simulink subsystem "PvtSubSys_PLAN_DPC"  (R2020b)
settings: Solver=VariableStepAuto  StartTime=0.0  StopTime=10.0  RelTol=1e-3
undefined symbols (not defined in the file or in its folder): P_Global_DxvFrontBumper_m, P_Global_DxvRearBumper_m, P_PLAN_DPC_BrkPointDxFactorF1, P_PLAN_DPC_BrkPointDxFactorF2, P_PLAN_DPC_BrkPointDxFactorF3, P_PLAN_DPC_BrkPointDxFactorF4, P_PLAN_DPC_BrkPointDxFactorR1, P_PLAN_DPC_BrkPointDxFactorR2, P_PLAN_DPC_BrkPointDxFactorR3, P_PLAN_DPC_BrkPointDxFactorR4, P_PLAN_DPC_danqianleida_kaiguan, P_PLAN_DPC_danqianleida_maxDx, P_PLAN_DPC_danqianleida_minDx, P_PLAN_DPC_FrontObj_DX_00, P_PLAN_DPC_FrontObj_DX_03, P_PLAN_DPC_FrontObj_DX_08, P_PLAN_DPC_FrontObj_DX_1, P_PLAN_DPC_HearObj_DX_00, P_PLAN_DPC_HearObj_DX_03, P_PLAN_DPC_HearObj_DX_08, P_PLAN_DPC_HearObj_DX_11, P_PLAN_DPC_HWALineRearA2Factor, P_PLAN_DPC_HWALineRearA3Factor, P_PLAN_DPC_ObjAxLPalpha, P_PLAN_DPC_ObjDxLPalpha, P_PLAN_DPC_ObjDyLPalpha, P_PLAN_DPC_ObjVxLPalpha, P_PLAN_DPC_xiangduisudu_kmh
libraries: simulink x22
(part 2 of 3)

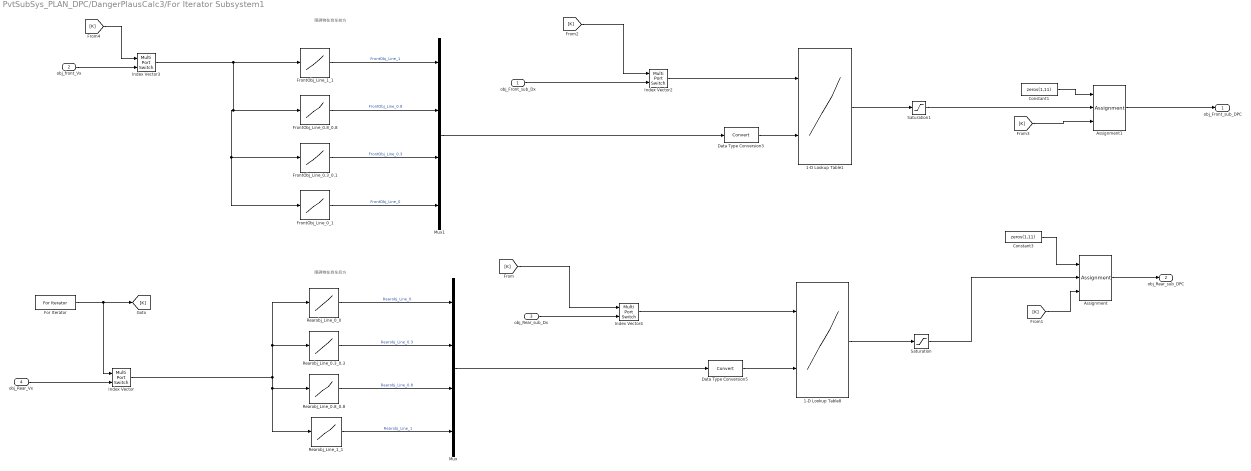
== system PvtSubSys_PLAN_DPC/DangerPlausCalc3/For Iterator Subsystem1 ==
  note: 障碍物在自车后方
  note: 障碍物在自车前方
  obj_Front_sub_Dx : Inport
  obj_front_Vx : Inport  Port=2
  obj_Rear_sub_Dx : Inport  Port=3
  obj_Rear_Vx : Inport  Port=4
  1-D Lookup Table1 : Lookup_n-D  NumberOfTableDimensions=1  BreakpointsForDimension1Source=Input port  BreakpointsForDimension1=[-5:5]  Table=[1 0.8 0.3 0]  InternalRulePriority=Speed  RndMeth=Simplest  InputSameDT=on
      settings: InputPortMap=u0,p5
  1-D Lookup Table8 : Lookup_n-D  NumberOfTableDimensions=1  BreakpointsForDimension1Source=Input port  BreakpointsForDimension1=[-5:5]  Table=[0 0.3 0.8 1]  InternalRulePriority=Speed  RndMeth=Simplest  InputSameDT=on
      settings: InputPortMap=u0,p5
  Assignment : Assignment  DiagnosticForDimensions=Warning  IndexOptions=Index vector (port)  Indices=1  OutputSizes=1
  Assignment1 : Assignment  DiagnosticForDimensions=Warning  IndexOptions=Index vector (port)  Indices=1  OutputSizes=1
  Constant1 : Constant  Value=zeros(1,11)  OutDataTypeStr=single
  Constant3 : Constant  Value=zeros(1,11)  OutDataTypeStr=single
  Data Type Conversion3 : DataTypeConversion
  Data Type Conversion5 : DataTypeConversion
  For Iterator : ForIterator  ResetStates=reset  IterationLimit=11  IterationVariableDataType=int8
  FrontObj_Line_0.3_0.1 : Lookup_n-D  NumberOfTableDimensions=1  BreakpointsForDimension1="[-49.5\t-33\t-18\t-16.5\t-7\t-6\t-2.5\t-2\t-1.5\t-0.5\t0\t0.5\t1.5\t4\t4.5\t5\t5.5\t7\t9.5\t10\t12.5\t18.5\t30]"  Table="[160\t112\t64\t60\t26.4\t23.6\t19\t18.4\t17.8\t16.6\t16.2\t15.6\t14.6\t13\t12.8\t12.4\t12.2\t11.8\t11.2\t11\t10.6\t9.2\t9.2]"  InternalRulePriority=Speed  RndMeth=Simplest  InputSameDT=on
  FrontObj_Line_0.8_0.8 : Lookup_n-D  NumberOfTableDimensions=1  BreakpointsForDimension1="[-49.5\t-33\t-18\t-16.5\t-7\t-6\t-2.5\t-2\t-1.5\t-0.5\t0\t0.5\t1.5\t4\t4.5\t5\t5.5\t7\t9.5\t10\t12.5\t18.5\t30]"  Table="[82\t58\t31.2\t29.2\t16\t14.8\t11\t10.4\t9.8\t8.6\t8.2\t7.6\t7.6\t7.6\t7.6\t7.6\t7.6\t7.6\t7.6\t7.6\t7.6\t7.6\t7.6]"  InternalRulePriority=Speed  RndMeth=Simplest  InputSameDT=on
  FrontObj_Line_0_1 : Lookup_n-D  NumberOfTableDimensions=1  BreakpointsForDimension1="[-49.5\t-33\t-18\t-16.5\t-7\t-6\t-2.5\t-2\t-1.5\t-0.5\t0\t0.5\t1.5\t4\t4.5\t5\t5.5\t7\t9.5\t10\t12.5\t18.5\t30]"  Table="[215\t150\t89\t82\t36.4\t32.4\t23.8\t23.2\t22.6\t21.6\t21\t20.4\t19.2\t16.6\t16\t15.4\t15.2\t14.4\t13.2\t13.2\t12.4\t11.2\t11.2]"  InternalRulePriority=Speed  RndMeth=Simplest  InputSameDT=on
  FrontObj_Line_1_1 : Lookup_n-D  NumberOfTableDimensions=1  BreakpointsForDimension1="[-49.5\t-33\t-18\t-16.5\t-7\t-6\t-2.5\t-2\t-1.5\t-0.5\t0\t0.5\t1.5\t4\t4.5\t5\t5.5\t7\t9.5\t10\t12.5\t18.5\t30]"  Table="[68\t46\t26.2\t24.4\t14\t12.8\t9\t8.4\t7.8\t6.6\t6.2\t5.6\t5.6\t5.6\t5.6\t5.6\t5.6\t5.6\t5.6\t5.6\t5.6\t5.6\t5.6]"  ExtrapMethod=Clip  UseLastTableValue=on  InternalRulePriority=Speed  RndMeth=Simplest  InputSameDT=on
  Index Vector : MultiPortSwitch  Inputs=1
  Index Vector2 : MultiPortSwitch  Inputs=1  OutDataTypeStr=single
  Index Vector3 : MultiPortSwitch  Inputs=1
  Index Vector4 : MultiPortSwitch  Inputs=1  OutDataTypeStr=single
  Mux : Mux
  Mux1 : Mux
  Rearobj_Line_0.3_0.3 : Lookup_n-D  NumberOfTableDimensions=1  BreakpointsForDimension1="[-49.5\t-33\t-18\t-16.5\t-7\t-6\t-2.5\t-2\t-1.5\t-0.5\t0\t0.5\t1.5\t4\t4.5\t5\t5.5\t7\t9.5\t10\t12.5\t18.5\t30]"  Table="[-2.7\t-3.4\t-4.6\t-4.8\t-6.6\t-7\t-8.8\t-9\t-9.4\t-10.2\t-10.8\t-11.2\t-12.4\t-15.2\t-15.6\t-16.2\t-16.8\t-18.4\t-24.2\t-25.6\t-32.4\t-48.5\t-76.4]"  InternalRulePriority=Speed  RndMeth=Simplest  InputSameDT=on
  Rearobj_Line_0.8_0.8 : Lookup_n-D  NumberOfTableDimensions=1  BreakpointsForDimension1="[-49.5\t-33\t-18\t-16.5\t-7\t-6\t-2.5\t-2\t-1.5\t-0.5\t0\t0.5\t1.5\t4\t4.5\t5\t5.5\t7\t9.5\t10\t12.5\t18.5\t30]"  Table="[-1.19\t-1.2\t-1.2\t-1.2\t-1.2\t-1.2\t-1.2\t-1.2\t-1.2\t-1.2\t-1.2\t-1.2\t-2.4\t-5.2\t-5.6\t-6.2\t-6.8\t-8.4\t-11.8\t-12.4\t-16\t-24.2\t-38]"  InternalRulePriority=Speed  RndMeth=Simplest  InputSameDT=on
  Rearobj_Line_0_0 : Lookup_n-D  NumberOfTableDimensions=1  BreakpointsForDimension1="[-49.5\t-33\t-18\t-16.5\t-7\t-6\t-2.5\t-2\t-1.5\t-0.5\t0\t0.5\t1.5\t4\t4.5\t5\t5.5\t7\t9.5\t10\t12.5\t18.5\t30]"  Table="[-3.9\t-5\t-7\t-7.4\t-11\t-11.8\t-15.6\t-16.2\t-16.8\t-17.8\t-18.4\t-19\t-20\t-22.8\t-23.4\t-24\t-24.6\t-28.2\t-38.2\t-40.2\t-47.3\t-71\t-100]"  InternalRulePriority=Speed  RndMeth=Simplest  InputSameDT=on
  Rearobj_Line_1_1 : Lookup_n-D  NumberOfTableDimensions=1  BreakpointsForDimension1="[-49.5\t-33\t-18\t-16.5\t-7\t-6\t-2.5\t-2\t-1.5\t-0.5\t0\t0.5\t1.5\t4\t4.5\t5\t5.5\t7\t9.5\t10\t12.5\t18.5\t30]"  Table="[0.8\t0.8\t0.8\t0.8\t0.8\t0.8\t0.8\t0.8\t0.8\t0.8\t0.8\t0.8\t-0.4\t-3.2\t-3.6\t-4.2\t-4.8\t-6.4\t-9.2\t-9.8\t-12.6\t-19.2\t-30]"  InternalRulePriority=Speed  RndMeth=Simplest  InputSameDT=on
  Saturation : Saturate  UpperLimit=1  LowerLimit=0
  Saturation1 : Saturate  UpperLimit=1  LowerLimit=0
  obj_Front_sub_DPC : Outport
  obj_Rear_sub_DPC : Outport  Port=2
  wires:
  Data Type Conversion5/1 -> 1-D Lookup Table8/2
  Index Vector4/1 -> 1-D Lookup Table8/1
  Data Type Conversion3/1 -> 1-D Lookup Table1/2
  Index Vector2/1 -> 1-D Lookup Table1/1
  Saturation/1 -> Assignment/2
  Saturation1/1 -> Assignment1/2
  obj_front_Vx/1 -> Index Vector3/2
  Index Vector3/1 -> FrontObj_Line_1_1/1, FrontObj_Line_0_1/1, FrontObj_Line_0.3_0.1/1, FrontObj_Line_0.8_0.8/1
  [K] -> Index Vector3/1
  Assignment1/1 -> obj_Front_sub_DPC/1
  Constant1/1 -> Assignment1/1
  [K] -> Assignment1/3
  [K] -> Index Vector2/1
  Assignment/1 -> obj_Rear_sub_DPC/1
  [K] -> Assignment/3
  Constant3/1 -> Assignment/1
  [K] -> Index Vector4/1
  For Iterator/1 -> [K], Index Vector/1
  obj_Rear_Vx/1 -> Index Vector/2
  Rearobj_Line_0.3_0.3/1 -> Mux/2  "Rearobj_Line_0.3"
  Index Vector/1 -> Rearobj_Line_0.3_0.3/1, Rearobj_Line_0_0/1, Rearobj_Line_1_1/1, Rearobj_Line_0.8_0.8/1
  Mux1/1 -> Data Type Conversion3/1
  FrontObj_Line_0.8_0.8/1 -> Mux1/2  "FrontObj_Line_0.8"
  obj_Front_sub_Dx/1 -> Index Vector2/2
  FrontObj_Line_1_1/1 -> Mux1/1  "FrontObj_Line_1"
  1-D Lookup Table1/1 -> Saturation1/1
  Rearobj_Line_1_1/1 -> Mux/4  "Rearobj_Line_1"
  FrontObj_Line_0_1/1 -> Mux1/4  "FrontObj_Line_0"
  1-D Lookup Table8/1 -> Saturation/1
  Mux/1 -> Data Type Conversion5/1
  obj_Rear_sub_Dx/1 -> Index Vector4/2
  Rearobj_Line_0_0/1 -> Mux/1  "Rearobj_Line_0"
  FrontObj_Line_0.3_0.1/1 -> Mux1/3  "FrontObj_Line_0.3"
  Rearobj_Line_0.8_0.8/1 -> Mux/3  "Rearobj_Line_0.8"

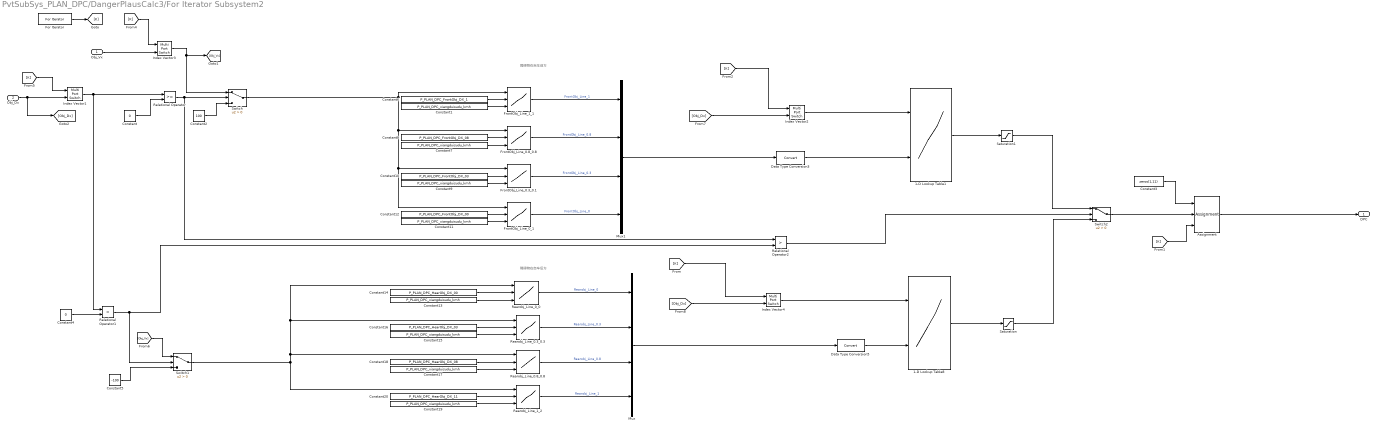
== system PvtSubSys_PLAN_DPC/DangerPlausCalc3/For Iterator Subsystem2 ==
  note: 障碍物在自车后方
  note: 障碍物在自车前方
  Obj_Vx : Inport
  Obj_Dx : Inport  Port=2
  1-D Lookup Table1 : Lookup_n-D  NumberOfTableDimensions=1  BreakpointsForDimension1Source=Input port  BreakpointsForDimension1=[-5:5]  Table=[1 0.8 0.3 0]  ExtrapMethod=Clip  InternalRulePriority=Speed  RndMeth=Simplest  InputSameDT=on
      settings: InputPortMap=u0,p5
  1-D Lookup Table8 : Lookup_n-D  NumberOfTableDimensions=1  BreakpointsForDimension1Source=Input port  BreakpointsForDimension1=[-5:5]  Table=[0 0.3 0.8 1]  ExtrapMethod=Clip  InternalRulePriority=Speed  RndMeth=Simplest  InputSameDT=on
      settings: InputPortMap=u0,p5
  Assignment : Assignment  DiagnosticForDimensions=Warning  IndexOptions=Index vector (port)  Indices=1  OutputSizes=1
  Constant : Constant  Value=0  OutDataTypeStr=single
  Constant{1,7,9,11,13,15,17,19} (8 alike) : Constant  Value=P_PLAN_DPC_xiangduisudu_kmh  OutDataTypeStr=single
  Constant10 : Constant  Value=P_PLAN_DPC_FrontObj_DX_03  OutDataTypeStr=single
  Constant12 : Constant  Value=P_PLAN_DPC_FrontObj_DX_00  OutDataTypeStr=single
  Constant14 : Constant  Value=P_PLAN_DPC_HearObj_DX_00  OutDataTypeStr=single
  Constant16 : Constant  Value=P_PLAN_DPC_HearObj_DX_03  OutDataTypeStr=single
  Constant18 : Constant  Value=P_PLAN_DPC_HearObj_DX_08  OutDataTypeStr=single
  Constant2 : Constant  Value=100  OutDataTypeStr=single
  Constant20 : Constant  Value=P_PLAN_DPC_HearObj_DX_11  OutDataTypeStr=single
  Constant3 : Constant  Value=zeros(1,11)  OutDataTypeStr=single
  Constant4 : Constant  Value=0  OutDataTypeStr=single
  Constant5 : Constant  Value=-100  OutDataTypeStr=single
  Constant6 : Constant  Value=P_PLAN_DPC_FrontObj_DX_1  OutDataTypeStr=single
  Constant8 : Constant  Value=P_PLAN_DPC_FrontObj_DX_08  OutDataTypeStr=single
  Data Type Conversion3 : DataTypeConversion
  Data Type Conversion5 : DataTypeConversion
  For Iterator : ForIterator  ResetStates=reset  IterationLimit=11  IterationVariableDataType=int8
  FrontObj_Line_0.3_0.1 : Lookup_n-D  NumberOfTableDimensions=1  BreakpointsForDimension1Source=Input port  BreakpointsForDimension1="[-49.5\t-33\t-18\t-16.5\t-7\t-6\t-2.5\t-2\t-1.5\t-0.5\t0\t0.5\t1.5\t4\t4.5\t5\t5.5\t7\t9.5\t10\t12.5\t18.5\t30 50]"  TableSource=Input port  Table="[160\t112\t64\t60\t26.4\t23.6\t19\t18.4\t17.8\t16.6\t16.2\t15.6\t14.6\t13\t12.8\t12.4\t12.2\t11.8\t11.2\t11\t10.6\t9.2\t9.2 9.2]"  InternalRulePriority=Speed  RndMeth=Simplest  InputSameDT=on
      settings: InputPortMap=u0,p221,p5
  FrontObj_Line_0.8_0.8 : Lookup_n-D  NumberOfTableDimensions=1  BreakpointsForDimension1Source=Input port  BreakpointsForDimension1="[-49.5\t-33\t-18\t-16.5\t-7\t-6\t-2.5\t-2\t-1.5\t-0.5\t0\t0.5\t1.5\t4\t4.5\t5\t5.5\t7\t9.5\t10\t12.5\t18.5\t30 50]"  TableSource=Input port  Table="[82\t58\t31.2\t29.2\t16\t14.8\t11\t10.4\t9.8\t8.6\t8.2\t7.6\t7.6\t7.6\t7.6\t7.6\t7.6\t7.6\t7.6\t7.6\t7.6\t7.6\t7.6 7.6]"  InternalRulePriority=Speed  RndMeth=Simplest  InputSameDT=on
      settings: InputPortMap=u0,p221,p5
  FrontObj_Line_0_1 : Lookup_n-D  NumberOfTableDimensions=1  BreakpointsForDimension1Source=Input port  BreakpointsForDimension1="[-49.5\t-33\t-18\t-16.5\t-7\t-6\t-2.5\t-2\t-1.5\t-0.5\t0\t0.5\t1.5\t4\t4.5\t5\t5.5\t7\t9.5\t10\t12.5\t18.5\t30 50]"  TableSource=Input port  Table="[215\t150\t89\t82\t36.4\t32.4\t23.8\t23.2\t22.6\t21.6\t21\t20.4\t19.2\t16.6\t16\t15.4\t15.2\t14.4\t13.2\t13.2\t12.4\t11.2\t11.2 11.2]"  InternalRulePriority=Speed  RndMeth=Simplest  InputSameDT=on
      settings: InputPortMap=u0,p221,p5
  FrontObj_Line_1_1 : Lookup_n-D  NumberOfTableDimensions=1  BreakpointsForDimension1Source=Input port  BreakpointsForDimension1="[-49.5\t-33\t-18\t-16.5\t-7\t-6\t-2.5\t-2\t-1.5\t-0.5\t0\t0.5\t1.5\t4\t4.5\t5\t5.5\t7\t9.5\t10\t12.5\t18.5\t30 50]"  TableSource=Input port  Table="[68\t      46\t26.2\t24.4\t14\t    12.8\t9\t    8.4 \t7.8\t     6.6\t6.2\t     5.6\t5.6 \t5.6\t     5.6\t5.6\t     5.6\t5.6\t    5.6\t    5.6     5.6\t     5.6\t5.6  5.6]"  UseLastTableValue=on  InternalRulePriority=Speed  RndMeth=Simplest  InputSameDT=on
      settings: InputPortMap=u0,p221,p5
  Index Vector1 : MultiPortSwitch  Inputs=1
  Index Vector2 : MultiPortSwitch  Inputs=1  OutDataTypeStr=single
  Index Vector3 : MultiPortSwitch  Inputs=1
  Index Vector4 : MultiPortSwitch  Inputs=1  OutDataTypeStr=single
  Mux : Mux
  Mux1 : Mux
  Rearobj_Line_0.3_0.3 : Lookup_n-D  NumberOfTableDimensions=1  BreakpointsForDimension1Source=Input port  BreakpointsForDimension1="[-49.5\t-33\t-18\t-16.5\t-7\t-6\t-2.5\t-2\t-1.5\t-0.5\t0\t0.5\t1.5\t4\t4.5\t5\t5.5\t7\t9.5\t10\t12.5\t18.5\t30 50]"  TableSource=Input port  Table="[-7   \t-7  \t-7  \t-7  \t-7  \t-7  \t -8.1 \t-9  \t-9.4  \t-10.2\t-10.8\t-11.2\t-12.4\t-15.2\t-15.6\t-16.2\t-16.8\t-19.4\t-24.2\t-25.6\t-30.4\t-48.5\t-86.4 -140]"  InternalRulePriority=Speed  RndMeth=Simplest  InputSameDT=on
      settings: InputPortMap=u0,p221,p5
  Rearobj_Line_0.8_0.8 : Lookup_n-D  NumberOfTableDimensions=1  BreakpointsForDimension1Source=Input port  BreakpointsForDimension1="[-49.5\t-33\t-18\t-16.5\t-7\t-6\t-2.5\t-2\t-1.5\t-0.5\t0\t0.5\t1.5\t4\t4.5\t5\t5.5\t7\t9.5\t10\t12.5\t18.5\t30 50]"  TableSource=Input port  Table="[-2.4    -2.4\t    -2.4\t-2.4\t-2.4\t-2.4\t-2.4\t-2.4\t-2.4\t-2.4\t-2.4\t-2.4\t-2.4\t-5.2\t-5.6\t-6.2\t  -6.8   \t-8.4\t-11.8\t-12.4\t-16\t    -24.2\t-38 -60]"  InternalRulePriority=Speed  RndMeth=Simplest  InputSameDT=on
      settings: InputPortMap=u0,p221,p5
  Rearobj_Line_0_0 : Lookup_n-D  NumberOfTableDimensions=1  BreakpointsForDimension1Source=Input port  BreakpointsForDimension1="[-49.5\t-33\t-18\t-16.5\t-7\t-6\t-2.5\t-2\t-1.5\t-0.5\t0\t0.5\t1.5\t4\t4.5\t5\t5.5\t7\t9.5\t10\t12.5\t18.5\t30 50]"  TableSource=Input port  Table="[-13\t     -13\t -13    -13 \t-13\t    -14\t    -15.6\t-16.2\t-16.8\t-17.8\t-18.4\t-19  \t-20  \t-22.8\t-23.4\t-24\t    -24.6\t-28.2\t-38.2\t-40.2\t-47.3\t-68\t    -100 -160]"  InternalRulePriority=Speed  RndMeth=Simplest  InputSameDT=on
      settings: InputPortMap=u0,p221,p5
  Rearobj_Line_1_2 : Lookup_n-D  NumberOfTableDimensions=1  BreakpointsForDimension1Source=Input port  BreakpointsForDimension1="[-49.5\t-33\t-18\t-16.5\t-7\t-6\t-2.5\t-2\t-1.5\t-0.5\t0\t0.5\t1.5\t4\t4.5\t5\t5.5\t7\t9.5\t10\t12.5\t18.5\t30 50]"  TableSource=Input port  Table="[-2\t     -2 \t-2\t    -2\t    -2 \t    -2    \t-2\t   -2 \t   -2\t    -2\t    -2      -2\t   -2       -3.2\t -3.6\t -4.2\t -4.8\t -6.4\t -9.2\t   -9.8\t   -12.6\t-19.2\t-30 -30]"  InternalRulePriority=Speed  RndMeth=Simplest  InputSameDT=on
      settings: InputPortMap=u0,p221,p5
  Relational Operator : RelationalOperator  OutDataTypeStr=boolean  RndMeth=Simplest
  Relational Operator1 : RelationalOperator  Operator=<  OutDataTypeStr=boolean  RndMeth=Simplest
  Relational Operator2 : RelationalOperator  Operator=>  OutDataTypeStr=boolean  RndMeth=Simplest
  Saturation : Saturate  UpperLimit=1  LowerLimit=0
  Saturation1 : Saturate  UpperLimit=1  LowerLimit=0
  Switch : Switch  Criteria=u2 > Threshold
  Switch1 : Switch  Criteria=u2 > Threshold
  Switch2 : Switch  Criteria=u2 > Threshold
  DPC : Outport
  wires:
  Constant19/1 -> Rearobj_Line_1_2/3
  Constant13/1 -> Rearobj_Line_0_0/3
  Constant18/1 -> Rearobj_Line_0.8_0.8/2
  Constant17/1 -> Rearobj_Line_0.8_0.8/3
  Constant14/1 -> Rearobj_Line_0_0/2
  Constant15/1 -> Rearobj_Line_0.3_0.3/3
  Switch1/1 -> Rearobj_Line_1_2/1, Rearobj_Line_0_0/1, Rearobj_Line_0.3_0.3/1, Rearobj_Line_0.8_0.8/1
  Constant20/1 -> Rearobj_Line_1_2/2
  Constant16/1 -> Rearobj_Line_0.3_0.3/2
  Switch/1 -> FrontObj_Line_0.8_0.8/1, FrontObj_Line_0.3_0.1/1, FrontObj_Line_0_1/1, FrontObj_Line_1_1/1
  Constant1/1 -> FrontObj_Line_1_1/3
  Constant8/1 -> FrontObj_Line_0.8_0.8/2
  Constant6/1 -> FrontObj_Line_1_1/2
  Constant9/1 -> FrontObj_Line_0.3_0.1/3
  Constant10/1 -> FrontObj_Line_0.3_0.1/2
  Constant11/1 -> FrontObj_Line_0_1/3
  Constant7/1 -> FrontObj_Line_0.8_0.8/3
  Constant12/1 -> FrontObj_Line_0_1/2
  Index Vector4/1 -> 1-D Lookup Table8/1
  Index Vector2/1 -> 1-D Lookup Table1/1
  Saturation/1 -> Switch2/3
  Saturation1/1 -> Switch2/1
  Switch2/1 -> Assignment/2
  Relational Operator2/1 -> Switch2/2
  Assignment/1 -> DPC/1
  [Obj_Dx] -> Index Vector4/2
  [Obj_Dx] -> Index Vector2/2
  Constant5/1 -> Switch1/3
  [Obj_Vx] -> Switch1/1
  Index Vector3/1 -> Switch/1, [Obj_Vx]
  Relational Operator1/1 -> Switch1/2, Relational Operator2/2
  Constant4/1 -> Relational Operator1/2
  Constant2/1 -> Switch/3
  Relational Operator/1 -> Switch/2, Relational Operator2/1
  Constant/1 -> Relational Operator/2
  Index Vector1/1 -> Relational Operator1/1, Relational Operator/1
  [K] -> Index Vector1/1
  Obj_Dx/1 -> Index Vector1/2, [Obj_Dx]
  Obj_Vx/1 -> Index Vector3/2
  Data Type Conversion5/1 -> 1-D Lookup Table8/2
  Data Type Conversion3/1 -> 1-D Lookup Table1/2
  [K] -> Index Vector3/1
  [K] -> Index Vector2/1
  [K] -> Assignment/3
  Constant3/1 -> Assignment/1
  [K] -> Index Vector4/1
  For Iterator/1 -> [K]
  Rearobj_Line_0.3_0.3/1 -> Mux/2  "Rearobj_Line_0.3"
  Mux1/1 -> Data Type Conversion3/1
  FrontObj_Line_0.8_0.8/1 -> Mux1/2  "FrontObj_Line_0.8"
  FrontObj_Line_1_1/1 -> Mux1/1  "FrontObj_Line_1"
  1-D Lookup Table1/1 -> Saturation1/1
  Rearobj_Line_1_2/1 -> Mux/4  "Rearobj_Line_1"
  FrontObj_Line_0_1/1 -> Mux1/4  "FrontObj_Line_0"
  1-D Lookup Table8/1 -> Saturation/1
  Mux/1 -> Data Type Conversion5/1
  Rearobj_Line_0_0/1 -> Mux/1  "Rearobj_Line_0"
  FrontObj_Line_0.3_0.1/1 -> Mux1/3  "FrontObj_Line_0.3"
  Rearobj_Line_0.8_0.8/1 -> Mux/3  "Rearobj_Line_0.8"

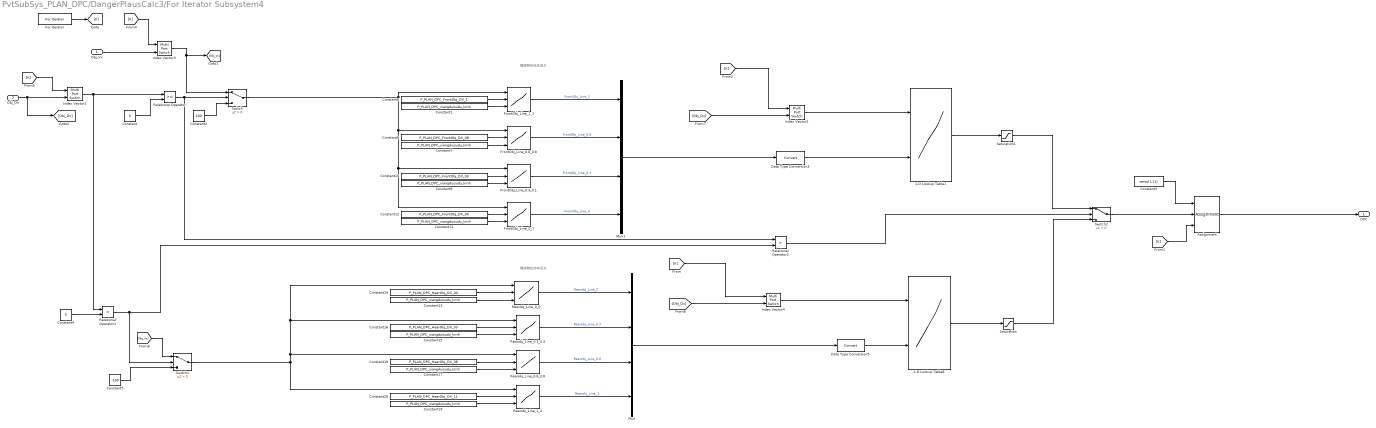
== system PvtSubSys_PLAN_DPC/DangerPlausCalc3/For Iterator Subsystem4 ==
  note: 障碍物在自车前方
  note: 障碍物在自车后方
  Obj_Vx : Inport
  Obj_Dx : Inport  Port=2
  1-D Lookup Table1 : Lookup_n-D  NumberOfTableDimensions=1  BreakpointsForDimension1Source=Input port  BreakpointsForDimension1=[-5:5]  Table=[1 0.8 0.3 0]  ExtrapMethod=Clip  InternalRulePriority=Speed  RndMeth=Simplest  InputSameDT=on
      settings: InputPortMap=u0,p5
  1-D Lookup Table8 : Lookup_n-D  NumberOfTableDimensions=1  BreakpointsForDimension1Source=Input port  BreakpointsForDimension1=[-5:5]  Table=[0 0.3 0.8 1]  ExtrapMethod=Clip  InternalRulePriority=Speed  RndMeth=Simplest  InputSameDT=on
      settings: InputPortMap=u0,p5
  Assignment : Assignment  DiagnosticForDimensions=Warning  IndexOptions=Index vector (port)  Indices=1  OutputSizes=1
  Constant : Constant  Value=0  OutDataTypeStr=single
  Constant{1,7,9,11,13,15,17,19} (8 alike) : Constant  Value=P_PLAN_DPC_xiangduisudu_kmh  OutDataTypeStr=single
  Constant10 : Constant  Value=P_PLAN_DPC_FrontObj_DX_03  OutDataTypeStr=single
  Constant12 : Constant  Value=P_PLAN_DPC_FrontObj_DX_00  OutDataTypeStr=single
  Constant14 : Constant  Value=P_PLAN_DPC_HearObj_DX_00  OutDataTypeStr=single
  Constant16 : Constant  Value=P_PLAN_DPC_HearObj_DX_03  OutDataTypeStr=single
  Constant18 : Constant  Value=P_PLAN_DPC_HearObj_DX_08  OutDataTypeStr=single
  Constant2 : Constant  Value=100  OutDataTypeStr=single
  Constant20 : Constant  Value=P_PLAN_DPC_HearObj_DX_11  OutDataTypeStr=single
  Constant3 : Constant  Value=zeros(1,11)  OutDataTypeStr=single
  Constant4 : Constant  Value=0  OutDataTypeStr=single
  Constant5 : Constant  Value=-100  OutDataTypeStr=single
  Constant6 : Constant  Value=P_PLAN_DPC_FrontObj_DX_1  OutDataTypeStr=single
  Constant8 : Constant  Value=P_PLAN_DPC_FrontObj_DX_08  OutDataTypeStr=single
  Data Type Conversion3 : DataTypeConversion
  Data Type Conversion5 : DataTypeConversion
  For Iterator : ForIterator  ResetStates=reset  IterationLimit=11  IterationVariableDataType=int8
  FrontObj_Line_0.3_0.1 : Lookup_n-D  NumberOfTableDimensions=1  BreakpointsForDimension1Source=Input port  BreakpointsForDimension1="[-49.5\t-33\t-18\t-16.5\t-7\t-6\t-2.5\t-2\t-1.5\t-0.5\t0\t0.5\t1.5\t4\t4.5\t5\t5.5\t7\t9.5\t10\t12.5\t18.5\t30 50]"  TableSource=Input port  Table="[160\t112\t64\t60\t26.4\t23.6\t19\t18.4\t17.8\t16.6\t16.2\t15.6\t14.6\t13\t12.8\t12.4\t12.2\t11.8\t11.2\t11\t10.6\t9.2\t9.2 9.2]"  InternalRulePriority=Speed  RndMeth=Simplest  InputSameDT=on
      settings: InputPortMap=u0,p221,p5
  FrontObj_Line_0.8_0.8 : Lookup_n-D  NumberOfTableDimensions=1  BreakpointsForDimension1Source=Input port  BreakpointsForDimension1="[-49.5\t-33\t-18\t-16.5\t-7\t-6\t-2.5\t-2\t-1.5\t-0.5\t0\t0.5\t1.5\t4\t4.5\t5\t5.5\t7\t9.5\t10\t12.5\t18.5\t30 50]"  TableSource=Input port  Table="[82\t58\t31.2\t29.2\t16\t14.8\t11\t10.4\t9.8\t8.6\t8.2\t7.6\t7.6\t7.6\t7.6\t7.6\t7.6\t7.6\t7.6\t7.6\t7.6\t7.6\t7.6 7.6]"  InternalRulePriority=Speed  RndMeth=Simplest  InputSameDT=on
      settings: InputPortMap=u0,p221,p5
  FrontObj_Line_0_1 : Lookup_n-D  NumberOfTableDimensions=1  BreakpointsForDimension1Source=Input port  BreakpointsForDimension1="[-49.5\t-33\t-18\t-16.5\t-7\t-6\t-2.5\t-2\t-1.5\t-0.5\t0\t0.5\t1.5\t4\t4.5\t5\t5.5\t7\t9.5\t10\t12.5\t18.5\t30 50]"  TableSource=Input port  Table="[215\t150\t89\t82\t36.4\t32.4\t23.8\t23.2\t22.6\t21.6\t21\t20.4\t19.2\t16.6\t16\t15.4\t15.2\t14.4\t13.2\t13.2\t12.4\t11.2\t11.2 11.2]"  InternalRulePriority=Speed  RndMeth=Simplest  InputSameDT=on
      settings: InputPortMap=u0,p221,p5
  FrontObj_Line_1_1 : Lookup_n-D  NumberOfTableDimensions=1  BreakpointsForDimension1Source=Input port  BreakpointsForDimension1="[-49.5\t-33\t-18\t-16.5\t-7\t-6\t-2.5\t-2\t-1.5\t-0.5\t0\t0.5\t1.5\t4\t4.5\t5\t5.5\t7\t9.5\t10\t12.5\t18.5\t30 50]"  TableSource=Input port  Table="[68\t      46\t26.2\t24.4\t14\t    12.8\t9\t    8.4 \t7.8\t     6.6\t6.2\t     5.6\t5.6 \t5.6\t     5.6\t5.6\t     5.6\t5.6\t    5.6\t    5.6     5.6\t     5.6\t5.6  5.6]"  UseLastTableValue=on  InternalRulePriority=Speed  RndMeth=Simplest  InputSameDT=on
      settings: InputPortMap=u0,p221,p5
  Index Vector1 : MultiPortSwitch  Inputs=1
  Index Vector2 : MultiPortSwitch  Inputs=1  OutDataTypeStr=single
  Index Vector3 : MultiPortSwitch  Inputs=1
  Index Vector4 : MultiPortSwitch  Inputs=1  OutDataTypeStr=single
  Mux : Mux
  Mux1 : Mux
  Rearobj_Line_0.3_0.3 : Lookup_n-D  NumberOfTableDimensions=1  BreakpointsForDimension1Source=Input port  BreakpointsForDimension1="[-49.5\t-33\t-18\t-16.5\t-7\t-6\t-2.5\t-2\t-1.5\t-0.5\t0\t0.5\t1.5\t4\t4.5\t5\t5.5\t7\t9.5\t10\t12.5\t18.5\t30 50]"  TableSource=Input port  Table="[-7   \t-7  \t-7  \t-7  \t-7  \t-7  \t -8.1 \t-9  \t-9.4  \t-10.2\t-10.8\t-11.2\t-12.4\t-15.2\t-15.6\t-16.2\t-16.8\t-19.4\t-24.2\t-25.6\t-30.4\t-48.5\t-86.4 -140]"  InternalRulePriority=Speed  RndMeth=Simplest  InputSameDT=on
      settings: InputPortMap=u0,p221,p5
  Rearobj_Line_0.8_0.8 : Lookup_n-D  NumberOfTableDimensions=1  BreakpointsForDimension1Source=Input port  BreakpointsForDimension1="[-49.5\t-33\t-18\t-16.5\t-7\t-6\t-2.5\t-2\t-1.5\t-0.5\t0\t0.5\t1.5\t4\t4.5\t5\t5.5\t7\t9.5\t10\t12.5\t18.5\t30 50]"  TableSource=Input port  Table="[-2.4    -2.4\t    -2.4\t-2.4\t-2.4\t-2.4\t-2.4\t-2.4\t-2.4\t-2.4\t-2.4\t-2.4\t-2.4\t-5.2\t-5.6\t-6.2\t  -6.8   \t-8.4\t-11.8\t-12.4\t-16\t    -24.2\t-38 -60]"  InternalRulePriority=Speed  RndMeth=Simplest  InputSameDT=on
      settings: InputPortMap=u0,p221,p5
  Rearobj_Line_0_0 : Lookup_n-D  NumberOfTableDimensions=1  BreakpointsForDimension1Source=Input port  BreakpointsForDimension1="[-49.5\t-33\t-18\t-16.5\t-7\t-6\t-2.5\t-2\t-1.5\t-0.5\t0\t0.5\t1.5\t4\t4.5\t5\t5.5\t7\t9.5\t10\t12.5\t18.5\t30 50]"  TableSource=Input port  Table="[-13\t     -13\t -13    -13 \t-13\t    -14\t    -15.6\t-16.2\t-16.8\t-17.8\t-18.4\t-19  \t-20  \t-22.8\t-23.4\t-24\t    -24.6\t-28.2\t-38.2\t-40.2\t-47.3\t-68\t    -100 -160]"  InternalRulePriority=Speed  RndMeth=Simplest  InputSameDT=on
      settings: InputPortMap=u0,p221,p5
  Rearobj_Line_1_2 : Lookup_n-D  NumberOfTableDimensions=1  BreakpointsForDimension1Source=Input port  BreakpointsForDimension1="[-49.5\t-33\t-18\t-16.5\t-7\t-6\t-2.5\t-2\t-1.5\t-0.5\t0\t0.5\t1.5\t4\t4.5\t5\t5.5\t7\t9.5\t10\t12.5\t18.5\t30 50]"  TableSource=Input port  Table="[-2\t     -2 \t-2\t    -2\t    -2 \t    -2    \t-2\t   -2 \t   -2\t    -2\t    -2      -2\t   -2       -3.2\t -3.6\t -4.2\t -4.8\t -6.4\t -9.2\t   -9.8\t   -12.6\t-19.2\t-30 -30]"  InternalRulePriority=Speed  RndMeth=Simplest  InputSameDT=on
      settings: InputPortMap=u0,p221,p5
  Relational Operator : RelationalOperator  OutDataTypeStr=boolean  RndMeth=Simplest
  Relational Operator1 : RelationalOperator  Operator=<  OutDataTypeStr=boolean  RndMeth=Simplest
  Relational Operator2 : RelationalOperator  Operator=>  OutDataTypeStr=boolean  RndMeth=Simplest
  Saturation : Saturate  UpperLimit=1  LowerLimit=0
  Saturation1 : Saturate  UpperLimit=1  LowerLimit=0
  Switch : Switch  Criteria=u2 > Threshold
  Switch1 : Switch  Criteria=u2 > Threshold
  Switch2 : Switch  Criteria=u2 > Threshold
  DPC : Outport
  wires:
  Rearobj_Line_0.8_0.8/1 -> Mux/3  "Rearobj_Line_0.8"
  FrontObj_Line_0.3_0.1/1 -> Mux1/3  "FrontObj_Line_0.3"
  Rearobj_Line_0_0/1 -> Mux/1  "Rearobj_Line_0"
  Mux/1 -> Data Type Conversion5/1
  1-D Lookup Table8/1 -> Saturation/1
  FrontObj_Line_0_1/1 -> Mux1/4  "FrontObj_Line_0"
  Rearobj_Line_1_2/1 -> Mux/4  "Rearobj_Line_1"
  1-D Lookup Table1/1 -> Saturation1/1
  FrontObj_Line_1_1/1 -> Mux1/1  "FrontObj_Line_1"
  FrontObj_Line_0.8_0.8/1 -> Mux1/2  "FrontObj_Line_0.8"
  Mux1/1 -> Data Type Conversion3/1
  Rearobj_Line_0.3_0.3/1 -> Mux/2  "Rearobj_Line_0.3"
  For Iterator/1 -> [K]
  [K] -> Index Vector4/1
  Constant3/1 -> Assignment/1
  [K] -> Assignment/3
  [K] -> Index Vector2/1
  [K] -> Index Vector3/1
  Data Type Conversion3/1 -> 1-D Lookup Table1/2
  Data Type Conversion5/1 -> 1-D Lookup Table8/2
  Obj_Vx/1 -> Index Vector3/2
  Obj_Dx/1 -> [Obj_Dx], Index Vector1/2
  [K] -> Index Vector1/1
  Index Vector1/1 -> Relational Operator/1, Relational Operator1/1
  Constant/1 -> Relational Operator/2
  Relational Operator/1 -> Relational Operator2/1, Switch/2
  Constant2/1 -> Switch/3
  Constant4/1 -> Relational Operator1/2
  Relational Operator1/1 -> Relational Operator2/2, Switch1/2
  Index Vector3/1 -> [Obj_Vx], Switch/1
  [Obj_Vx] -> Switch1/1
  Constant5/1 -> Switch1/3
  [Obj_Dx] -> Index Vector2/2
  [Obj_Dx] -> Index Vector4/2
  Assignment/1 -> DPC/1
  Relational Operator2/1 -> Switch2/2
  Switch2/1 -> Assignment/2
  Saturation1/1 -> Switch2/1
  Saturation/1 -> Switch2/3
  Index Vector2/1 -> 1-D Lookup Table1/1
  Index Vector4/1 -> 1-D Lookup Table8/1
  Constant12/1 -> FrontObj_Line_0_1/2
  Constant7/1 -> FrontObj_Line_0.8_0.8/3
  Constant11/1 -> FrontObj_Line_0_1/3
  Constant10/1 -> FrontObj_Line_0.3_0.1/2
  Constant9/1 -> FrontObj_Line_0.3_0.1/3
  Constant6/1 -> FrontObj_Line_1_1/2
  Constant8/1 -> FrontObj_Line_0.8_0.8/2
  Constant1/1 -> FrontObj_Line_1_1/3
  Switch/1 -> FrontObj_Line_1_1/1, FrontObj_Line_0_1/1, FrontObj_Line_0.3_0.1/1, FrontObj_Line_0.8_0.8/1
  Constant16/1 -> Rearobj_Line_0.3_0.3/2
  Constant20/1 -> Rearobj_Line_1_2/2
  Switch1/1 -> Rearobj_Line_0.8_0.8/1, Rearobj_Line_0.3_0.3/1, Rearobj_Line_0_0/1, Rearobj_Line_1_2/1
  Constant15/1 -> Rearobj_Line_0.3_0.3/3
  Constant14/1 -> Rearobj_Line_0_0/2
  Constant17/1 -> Rearobj_Line_0.8_0.8/3
  Constant18/1 -> Rearobj_Line_0.8_0.8/2
  Constant13/1 -> Rearobj_Line_0_0/3
  Constant19/1 -> Rearobj_Line_1_2/3

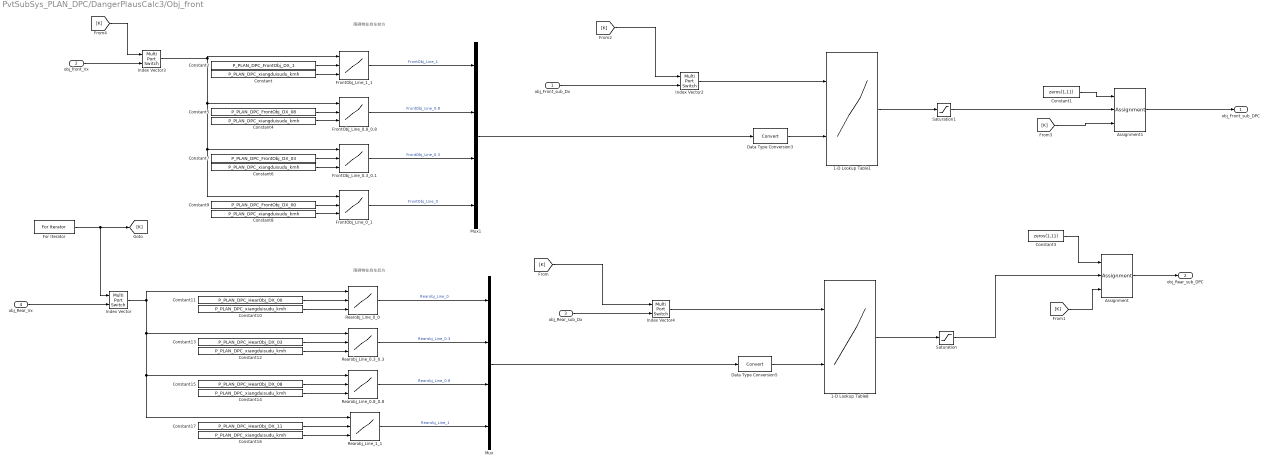
== system PvtSubSys_PLAN_DPC/DangerPlausCalc3/Obj_front ==
  note: 障碍物在自车前方
  note: 障碍物在自车后方
  obj_Front_sub_Dx : Inport
  obj_front_Vx : Inport  Port=2
  obj_Rear_sub_Dx : Inport  Port=3
  obj_Rear_Vx : Inport  Port=4
  1-D Lookup Table1 : Lookup_n-D  NumberOfTableDimensions=1  BreakpointsForDimension1Source=Input port  BreakpointsForDimension1=[-5:5]  Table=[1 0.8 0.3 0]  InternalRulePriority=Speed  RndMeth=Simplest  InputSameDT=on
      settings: InputPortMap=u0,p5
  1-D Lookup Table8 : Lookup_n-D  NumberOfTableDimensions=1  BreakpointsForDimension1Source=Input port  BreakpointsForDimension1=[-5:5]  Table=[0 0.3 0.8 1]  InternalRulePriority=Speed  RndMeth=Simplest  InputSameDT=on
      settings: InputPortMap=u0,p5
  Assignment : Assignment  DiagnosticForDimensions=Warning  IndexOptions=Index vector (port)  Indices=1  OutputSizes=1
  Assignment1 : Assignment  DiagnosticForDimensions=Warning  IndexOptions=Index vector (port)  Indices=1  OutputSizes=1
  Constant{,4,6,8,10,12,14,16} (8 alike) : Constant  Value=P_PLAN_DPC_xiangduisudu_kmh  OutDataTypeStr=single
  Constant1 : Constant  Value=zeros(1,11)  OutDataTypeStr=single
  Constant11 : Constant  Value=P_PLAN_DPC_HearObj_DX_00  OutDataTypeStr=single
  Constant13 : Constant  Value=P_PLAN_DPC_HearObj_DX_03  OutDataTypeStr=single
  Constant15 : Constant  Value=P_PLAN_DPC_HearObj_DX_08  OutDataTypeStr=single
  Constant17 : Constant  Value=P_PLAN_DPC_HearObj_DX_11  OutDataTypeStr=single
  Constant2 : Constant  Value=P_PLAN_DPC_FrontObj_DX_1  OutDataTypeStr=single
  Constant3 : Constant  Value=zeros(1,11)  OutDataTypeStr=single
  Constant5 : Constant  Value=P_PLAN_DPC_FrontObj_DX_08  OutDataTypeStr=single
  Constant7 : Constant  Value=P_PLAN_DPC_FrontObj_DX_03  OutDataTypeStr=single
  Constant9 : Constant  Value=P_PLAN_DPC_FrontObj_DX_00  OutDataTypeStr=single
  Data Type Conversion3 : DataTypeConversion
  Data Type Conversion5 : DataTypeConversion
  For Iterator : ForIterator  ResetStates=reset  IterationLimit=11  IterationVariableDataType=int8
  FrontObj_Line_0.3_0.1 : Lookup_n-D  NumberOfTableDimensions=1  BreakpointsForDimension1Source=Input port  BreakpointsForDimension1="[-49.5\t-33\t-18\t-16.5\t-7\t-6\t-2.5\t-2\t-1.5\t-0.5\t0\t0.5\t1.5\t4\t4.5\t5\t5.5\t7\t9.5\t10\t12.5\t18.5\t30 50]"  TableSource=Input port  Table="[160\t112\t64\t60\t26.4\t23.6\t19\t18.4\t17.8\t16.6\t16.2\t15.6\t14.6\t13\t12.8\t12.4\t12.2\t11.8\t11.2\t11\t10.6\t9.2\t9.2 9.2]"  InternalRulePriority=Speed  RndMeth=Simplest  InputSameDT=on
      settings: InputPortMap=u0,p221,p5
  FrontObj_Line_0.8_0.8 : Lookup_n-D  NumberOfTableDimensions=1  BreakpointsForDimension1Source=Input port  BreakpointsForDimension1="[-49.5\t-33\t-18\t-16.5\t-7\t-6\t-2.5\t-2\t-1.5\t-0.5\t0\t0.5\t1.5\t4\t4.5\t5\t5.5\t7\t9.5\t10\t12.5\t18.5\t30 50]"  TableSource=Input port  Table="[82\t58\t31.2\t29.2\t16\t14.8\t11\t10.4\t9.8\t8.6\t8.2\t7.6\t7.6\t7.6\t7.6\t7.6\t7.6\t7.6\t7.6\t7.6\t7.6\t7.6\t7.6 7.6]"  InternalRulePriority=Speed  RndMeth=Simplest  InputSameDT=on
      settings: InputPortMap=u0,p221,p5
  FrontObj_Line_0_1 : Lookup_n-D  NumberOfTableDimensions=1  BreakpointsForDimension1Source=Input port  BreakpointsForDimension1="[-49.5\t-33\t-18\t-16.5\t-7\t-6\t-2.5\t-2\t-1.5\t-0.5\t0\t0.5\t1.5\t4\t4.5\t5\t5.5\t7\t9.5\t10\t12.5\t18.5\t30 50]"  TableSource=Input port  Table="[215\t150\t89\t82\t36.4\t32.4\t23.8\t23.2\t22.6\t21.6\t21\t20.4\t19.2\t16.6\t16\t15.4\t15.2\t14.4\t13.2\t13.2\t12.4\t11.2\t11.2 11.2]"  InternalRulePriority=Speed  RndMeth=Simplest  InputSameDT=on
      settings: InputPortMap=u0,p221,p5
  FrontObj_Line_1_1 : Lookup_n-D  NumberOfTableDimensions=1  BreakpointsForDimension1Source=Input port  BreakpointsForDimension1="[-49.5\t-33\t-18\t-16.5\t-7\t-6\t-2.5\t-2\t-1.5\t-0.5\t0\t0.5\t1.5\t4\t4.5\t5\t5.5\t7\t9.5\t10\t12.5\t18.5\t30 50]"  TableSource=Input port  Table="[68\t      46\t26.2\t24.4\t14\t    12.8\t9\t    8.4 \t7.8\t     6.6\t6.2\t     5.6\t5.6 \t5.6\t     5.6\t5.6\t     5.6\t5.6\t    5.6\t    5.6     5.6\t     5.6\t5.6  5.6]"  UseLastTableValue=on  InternalRulePriority=Speed  RndMeth=Simplest  InputSameDT=on
      settings: InputPortMap=u0,p221,p5
  Index Vector : MultiPortSwitch  Inputs=1
  Index Vector2 : MultiPortSwitch  Inputs=1  OutDataTypeStr=single
  Index Vector3 : MultiPortSwitch  Inputs=1
  Index Vector4 : MultiPortSwitch  Inputs=1  OutDataTypeStr=single
  Mux : Mux
  Mux1 : Mux
  Rearobj_Line_0.3_0.3 : Lookup_n-D  NumberOfTableDimensions=1  BreakpointsForDimension1Source=Input port  BreakpointsForDimension1="[-49.5\t-33\t-18\t-16.5\t-7\t-6\t-2.5\t-2\t-1.5\t-0.5\t0\t0.5\t1.5\t4\t4.5\t5\t5.5\t7\t9.5\t10\t12.5\t18.5\t30 50]"  TableSource=Input port  Table="[-7   \t-7  \t-7  \t-7  \t-7  \t-7  \t -8.1 \t-9  \t-9.4  \t-10.2\t-10.8\t-11.2\t-12.4\t-15.2\t-15.6\t-16.2\t-16.8\t-19.4\t-24.2\t-25.6\t-30.4\t-48.5\t-86.4 -140]"  InternalRulePriority=Speed  RndMeth=Simplest  InputSameDT=on
      settings: InputPortMap=u0,p221,p5
  Rearobj_Line_0.8_0.8 : Lookup_n-D  NumberOfTableDimensions=1  BreakpointsForDimension1Source=Input port  BreakpointsForDimension1="[-49.5\t-33\t-18\t-16.5\t-7\t-6\t-2.5\t-2\t-1.5\t-0.5\t0\t0.5\t1.5\t4\t4.5\t5\t5.5\t7\t9.5\t10\t12.5\t18.5\t30 50]"  TableSource=Input port  Table="[-2.4    -2.4\t    -2.4\t-2.4\t-2.4\t-2.4\t-2.4\t-2.4\t-2.4\t-2.4\t-2.4\t-2.4\t-2.4\t-5.2\t-5.6\t-6.2\t  -6.8   \t-8.4\t-11.8\t-12.4\t-16\t    -24.2\t-38 -60]"  InternalRulePriority=Speed  RndMeth=Simplest  InputSameDT=on
      settings: InputPortMap=u0,p221,p5
  Rearobj_Line_0_0 : Lookup_n-D  NumberOfTableDimensions=1  BreakpointsForDimension1Source=Input port  BreakpointsForDimension1="[-49.5\t-33\t-18\t-16.5\t-7\t-6\t-2.5\t-2\t-1.5\t-0.5\t0\t0.5\t1.5\t4\t4.5\t5\t5.5\t7\t9.5\t10\t12.5\t18.5\t30 50]"  TableSource=Input port  Table="[-13\t     -13\t -13    -13 \t-13\t    -14\t    -15.6\t-16.2\t-16.8\t-17.8\t-18.4\t-19  \t-20  \t-22.8\t-23.4\t-24\t    -24.6\t-28.2\t-38.2\t-40.2\t-47.3\t-68\t    -100 -160]"  InternalRulePriority=Speed  RndMeth=Simplest  InputSameDT=on
      settings: InputPortMap=u0,p221,p5
  Rearobj_Line_1_1 : Lookup_n-D  NumberOfTableDimensions=1  BreakpointsForDimension1Source=Input port  BreakpointsForDimension1="[-49.5\t-33\t-18\t-16.5\t-7\t-6\t-2.5\t-2\t-1.5\t-0.5\t0\t0.5\t1.5\t4\t4.5\t5\t5.5\t7\t9.5\t10\t12.5\t18.5\t30 50]"  TableSource=Input port  Table="[-2\t     -2 \t-2\t    -2\t    -2 \t    -2    \t-2\t   -2 \t   -2\t    -2\t    -2      -2\t   -2       -3.2\t -3.6\t -4.2\t -4.8\t -6.4\t -9.2\t   -9.8\t   -12.6\t-19.2\t-30 -30]"  InternalRulePriority=Speed  RndMeth=Simplest  InputSameDT=on
      settings: InputPortMap=u0,p221,p5
  Saturation : Saturate  UpperLimit=1  LowerLimit=0
  Saturation1 : Saturate  UpperLimit=1  LowerLimit=0
  obj_Front_sub_DPC : Outport
  obj_Rear_sub_DPC : Outport  Port=2
  wires:
  Constant16/1 -> Rearobj_Line_1_1/3
  Constant17/1 -> Rearobj_Line_1_1/2
  Constant15/1 -> Rearobj_Line_0.8_0.8/2
  Constant14/1 -> Rearobj_Line_0.8_0.8/3
  Constant12/1 -> Rearobj_Line_0.3_0.3/3
  Constant13/1 -> Rearobj_Line_0.3_0.3/2
  Constant10/1 -> Rearobj_Line_0_0/3
  Constant11/1 -> Rearobj_Line_0_0/2
  Constant9/1 -> FrontObj_Line_0_1/2
  Constant8/1 -> FrontObj_Line_0_1/3
  Constant7/1 -> FrontObj_Line_0.3_0.1/2
  Constant6/1 -> FrontObj_Line_0.3_0.1/3
  Constant5/1 -> FrontObj_Line_0.8_0.8/2
  Constant4/1 -> FrontObj_Line_0.8_0.8/3
  Constant2/1 -> FrontObj_Line_1_1/2
  Constant/1 -> FrontObj_Line_1_1/3
  Rearobj_Line_0.8_0.8/1 -> Mux/3  "Rearobj_Line_0.8"
  FrontObj_Line_0.3_0.1/1 -> Mux1/3  "FrontObj_Line_0.3"
  Rearobj_Line_0_0/1 -> Mux/1  "Rearobj_Line_0"
  obj_Rear_sub_Dx/1 -> Index Vector4/2
  Mux/1 -> Data Type Conversion5/1
  1-D Lookup Table8/1 -> Saturation/1
  FrontObj_Line_0_1/1 -> Mux1/4  "FrontObj_Line_0"
  Rearobj_Line_1_1/1 -> Mux/4  "Rearobj_Line_1"
  1-D Lookup Table1/1 -> Saturation1/1
  FrontObj_Line_1_1/1 -> Mux1/1  "FrontObj_Line_1"
  obj_Front_sub_Dx/1 -> Index Vector2/2
  FrontObj_Line_0.8_0.8/1 -> Mux1/2  "FrontObj_Line_0.8"
  Mux1/1 -> Data Type Conversion3/1
  Index Vector/1 -> Rearobj_Line_0.3_0.3/1, Rearobj_Line_0.8_0.8/1, Rearobj_Line_1_1/1, Rearobj_Line_0_0/1
  Rearobj_Line_0.3_0.3/1 -> Mux/2  "Rearobj_Line_0.3"
  obj_Rear_Vx/1 -> Index Vector/2
  For Iterator/1 -> Index Vector/1, [K]
  [K] -> Index Vector4/1
  Constant3/1 -> Assignment/1
  [K] -> Assignment/3
  Assignment/1 -> obj_Rear_sub_DPC/1
  [K] -> Index Vector2/1
  [K] -> Assignment1/3
  Constant1/1 -> Assignment1/1
  Assignment1/1 -> obj_Front_sub_DPC/1
  [K] -> Index Vector3/1
  Index Vector3/1 -> FrontObj_Line_0.8_0.8/1, FrontObj_Line_0.3_0.1/1, FrontObj_Line_0_1/1, FrontObj_Line_1_1/1
  obj_front_Vx/1 -> Index Vector3/2
  Saturation1/1 -> Assignment1/2
  Saturation/1 -> Assignment/2
  Index Vector2/1 -> 1-D Lookup Table1/1
  Data Type Conversion3/1 -> 1-D Lookup Table1/2
  Index Vector4/1 -> 1-D Lookup Table8/1
  Data Type Conversion5/1 -> 1-D Lookup Table8/2

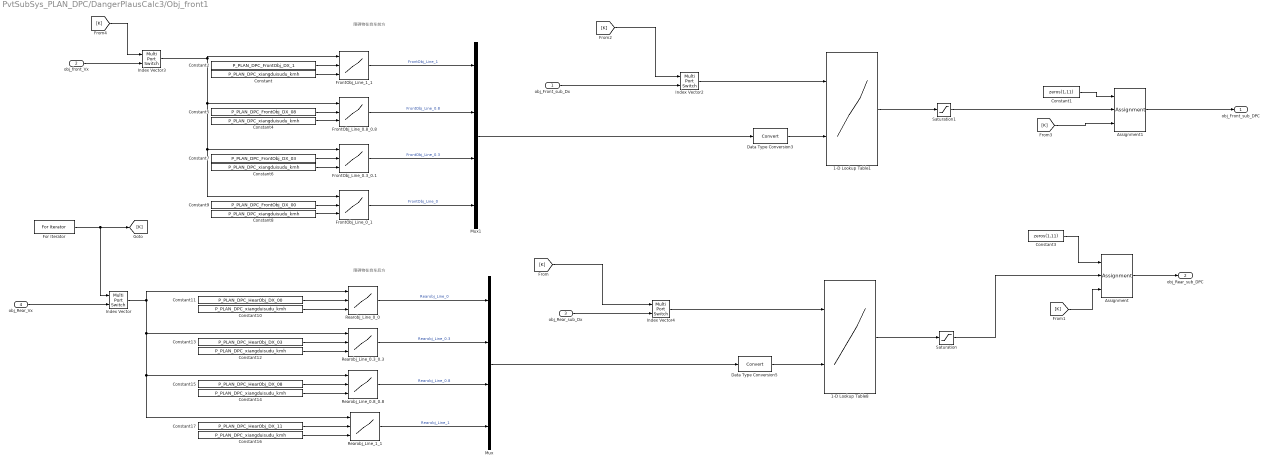
== system PvtSubSys_PLAN_DPC/DangerPlausCalc3/Obj_front1 ==
  note: 障碍物在自车后方
  note: 障碍物在自车前方
  obj_Front_sub_Dx : Inport
  obj_front_Vx : Inport  Port=2
  obj_Rear_sub_Dx : Inport  Port=3
  obj_Rear_Vx : Inport  Port=4
  1-D Lookup Table1 : Lookup_n-D  NumberOfTableDimensions=1  BreakpointsForDimension1Source=Input port  BreakpointsForDimension1=[-5:5]  Table=[1 0.8 0.3 0]  InternalRulePriority=Speed  RndMeth=Simplest  InputSameDT=on
      settings: InputPortMap=u0,p5
  1-D Lookup Table8 : Lookup_n-D  NumberOfTableDimensions=1  BreakpointsForDimension1Source=Input port  BreakpointsForDimension1=[-5:5]  Table=[0 0.3 0.8 1]  InternalRulePriority=Speed  RndMeth=Simplest  InputSameDT=on
      settings: InputPortMap=u0,p5
  Assignment : Assignment  DiagnosticForDimensions=Warning  IndexOptions=Index vector (port)  Indices=1  OutputSizes=1
  Assignment1 : Assignment  DiagnosticForDimensions=Warning  IndexOptions=Index vector (port)  Indices=1  OutputSizes=1
  Constant{,4,6,8,10,12,14,16} (8 alike) : Constant  Value=P_PLAN_DPC_xiangduisudu_kmh  OutDataTypeStr=single
  Constant1 : Constant  Value=zeros(1,11)  OutDataTypeStr=single
  Constant11 : Constant  Value=P_PLAN_DPC_HearObj_DX_00  OutDataTypeStr=single
  Constant13 : Constant  Value=P_PLAN_DPC_HearObj_DX_03  OutDataTypeStr=single
  Constant15 : Constant  Value=P_PLAN_DPC_HearObj_DX_08  OutDataTypeStr=single
  Constant17 : Constant  Value=P_PLAN_DPC_HearObj_DX_11  OutDataTypeStr=single
  Constant2 : Constant  Value=P_PLAN_DPC_FrontObj_DX_1  OutDataTypeStr=single
  Constant3 : Constant  Value=zeros(1,11)  OutDataTypeStr=single
  Constant5 : Constant  Value=P_PLAN_DPC_FrontObj_DX_08  OutDataTypeStr=single
  Constant7 : Constant  Value=P_PLAN_DPC_FrontObj_DX_03  OutDataTypeStr=single
  Constant9 : Constant  Value=P_PLAN_DPC_FrontObj_DX_00  OutDataTypeStr=single
  Data Type Conversion3 : DataTypeConversion
  Data Type Conversion5 : DataTypeConversion
  For Iterator : ForIterator  ResetStates=reset  IterationLimit=11  IterationVariableDataType=int8
  FrontObj_Line_0.3_0.1 : Lookup_n-D  NumberOfTableDimensions=1  BreakpointsForDimension1Source=Input port  BreakpointsForDimension1="[-49.5\t-33\t-18\t-16.5\t-7\t-6\t-2.5\t-2\t-1.5\t-0.5\t0\t0.5\t1.5\t4\t4.5\t5\t5.5\t7\t9.5\t10\t12.5\t18.5\t30 50]"  TableSource=Input port  Table="[160\t112\t64\t60\t26.4\t23.6\t19\t18.4\t17.8\t16.6\t16.2\t15.6\t14.6\t13\t12.8\t12.4\t12.2\t11.8\t11.2\t11\t10.6\t9.2\t9.2 9.2]"  InternalRulePriority=Speed  RndMeth=Simplest  InputSameDT=on
      settings: InputPortMap=u0,p221,p5
  FrontObj_Line_0.8_0.8 : Lookup_n-D  NumberOfTableDimensions=1  BreakpointsForDimension1Source=Input port  BreakpointsForDimension1="[-49.5\t-33\t-18\t-16.5\t-7\t-6\t-2.5\t-2\t-1.5\t-0.5\t0\t0.5\t1.5\t4\t4.5\t5\t5.5\t7\t9.5\t10\t12.5\t18.5\t30 50]"  TableSource=Input port  Table="[82\t58\t31.2\t29.2\t16\t14.8\t11\t10.4\t9.8\t8.6\t8.2\t7.6\t7.6\t7.6\t7.6\t7.6\t7.6\t7.6\t7.6\t7.6\t7.6\t7.6\t7.6 7.6]"  InternalRulePriority=Speed  RndMeth=Simplest  InputSameDT=on
      settings: InputPortMap=u0,p221,p5
  FrontObj_Line_0_1 : Lookup_n-D  NumberOfTableDimensions=1  BreakpointsForDimension1Source=Input port  BreakpointsForDimension1="[-49.5\t-33\t-18\t-16.5\t-7\t-6\t-2.5\t-2\t-1.5\t-0.5\t0\t0.5\t1.5\t4\t4.5\t5\t5.5\t7\t9.5\t10\t12.5\t18.5\t30 50]"  TableSource=Input port  Table="[215\t150\t89\t82\t36.4\t32.4\t23.8\t23.2\t22.6\t21.6\t21\t20.4\t19.2\t16.6\t16\t15.4\t15.2\t14.4\t13.2\t13.2\t12.4\t11.2\t11.2 11.2]"  InternalRulePriority=Speed  RndMeth=Simplest  InputSameDT=on
      settings: InputPortMap=u0,p221,p5
  FrontObj_Line_1_1 : Lookup_n-D  NumberOfTableDimensions=1  BreakpointsForDimension1Source=Input port  BreakpointsForDimension1="[-49.5\t-33\t-18\t-16.5\t-7\t-6\t-2.5\t-2\t-1.5\t-0.5\t0\t0.5\t1.5\t4\t4.5\t5\t5.5\t7\t9.5\t10\t12.5\t18.5\t30 50]"  TableSource=Input port  Table="[68\t      46\t26.2\t24.4\t14\t    12.8\t9\t    8.4 \t7.8\t     6.6\t6.2\t     5.6\t5.6 \t5.6\t     5.6\t5.6\t     5.6\t5.6\t    5.6\t    5.6     5.6\t     5.6\t5.6  5.6]"  UseLastTableValue=on  InternalRulePriority=Speed  RndMeth=Simplest  InputSameDT=on
      settings: InputPortMap=u0,p221,p5
  Index Vector : MultiPortSwitch  Inputs=1
  Index Vector2 : MultiPortSwitch  Inputs=1  OutDataTypeStr=single
  Index Vector3 : MultiPortSwitch  Inputs=1
  Index Vector4 : MultiPortSwitch  Inputs=1  OutDataTypeStr=single
  Mux : Mux
  Mux1 : Mux
  Rearobj_Line_0.3_0.3 : Lookup_n-D  NumberOfTableDimensions=1  BreakpointsForDimension1Source=Input port  BreakpointsForDimension1="[-49.5\t-33\t-18\t-16.5\t-7\t-6\t-2.5\t-2\t-1.5\t-0.5\t0\t0.5\t1.5\t4\t4.5\t5\t5.5\t7\t9.5\t10\t12.5\t18.5\t30 50]"  TableSource=Input port  Table="[-7   \t-7  \t-7  \t-7  \t-7  \t-7  \t -8.1 \t-9  \t-9.4  \t-10.2\t-10.8\t-11.2\t-12.4\t-15.2\t-15.6\t-16.2\t-16.8\t-19.4\t-24.2\t-25.6\t-30.4\t-48.5\t-86.4 -140]"  InternalRulePriority=Speed  RndMeth=Simplest  InputSameDT=on
      settings: InputPortMap=u0,p221,p5
  Rearobj_Line_0.8_0.8 : Lookup_n-D  NumberOfTableDimensions=1  BreakpointsForDimension1Source=Input port  BreakpointsForDimension1="[-49.5\t-33\t-18\t-16.5\t-7\t-6\t-2.5\t-2\t-1.5\t-0.5\t0\t0.5\t1.5\t4\t4.5\t5\t5.5\t7\t9.5\t10\t12.5\t18.5\t30 50]"  TableSource=Input port  Table="[-2.4    -2.4\t    -2.4\t-2.4\t-2.4\t-2.4\t-2.4\t-2.4\t-2.4\t-2.4\t-2.4\t-2.4\t-2.4\t-5.2\t-5.6\t-6.2\t  -6.8   \t-8.4\t-11.8\t-12.4\t-16\t    -24.2\t-38 -60]"  InternalRulePriority=Speed  RndMeth=Simplest  InputSameDT=on
      settings: InputPortMap=u0,p221,p5
  Rearobj_Line_0_0 : Lookup_n-D  NumberOfTableDimensions=1  BreakpointsForDimension1Source=Input port  BreakpointsForDimension1="[-49.5\t-33\t-18\t-16.5\t-7\t-6\t-2.5\t-2\t-1.5\t-0.5\t0\t0.5\t1.5\t4\t4.5\t5\t5.5\t7\t9.5\t10\t12.5\t18.5\t30 50]"  TableSource=Input port  Table="[-13\t     -13\t -13    -13 \t-13\t    -14\t    -15.6\t-16.2\t-16.8\t-17.8\t-18.4\t-19  \t-20  \t-22.8\t-23.4\t-24\t    -24.6\t-28.2\t-38.2\t-40.2\t-47.3\t-68\t    -100 -160]"  InternalRulePriority=Speed  RndMeth=Simplest  InputSameDT=on
      settings: InputPortMap=u0,p221,p5
  Rearobj_Line_1_1 : Lookup_n-D  NumberOfTableDimensions=1  BreakpointsForDimension1Source=Input port  BreakpointsForDimension1="[-49.5\t-33\t-18\t-16.5\t-7\t-6\t-2.5\t-2\t-1.5\t-0.5\t0\t0.5\t1.5\t4\t4.5\t5\t5.5\t7\t9.5\t10\t12.5\t18.5\t30 50]"  TableSource=Input port  Table="[-2\t     -2 \t-2\t    -2\t    -2 \t    -2    \t-2\t   -2 \t   -2\t    -2\t    -2      -2\t   -2       -3.2\t -3.6\t -4.2\t -4.8\t -6.4\t -9.2\t   -9.8\t   -12.6\t-19.2\t-30 -30]"  InternalRulePriority=Speed  RndMeth=Simplest  InputSameDT=on
      settings: InputPortMap=u0,p221,p5
  Saturation : Saturate  UpperLimit=1  LowerLimit=0
  Saturation1 : Saturate  UpperLimit=1  LowerLimit=0
  obj_Front_sub_DPC : Outport
  obj_Rear_sub_DPC : Outport  Port=2
  wires:
  Data Type Conversion5/1 -> 1-D Lookup Table8/2
  Index Vector4/1 -> 1-D Lookup Table8/1
  Data Type Conversion3/1 -> 1-D Lookup Table1/2
  Index Vector2/1 -> 1-D Lookup Table1/1
  Saturation/1 -> Assignment/2
  Saturation1/1 -> Assignment1/2
  obj_front_Vx/1 -> Index Vector3/2
  Index Vector3/1 -> FrontObj_Line_1_1/1, FrontObj_Line_0_1/1, FrontObj_Line_0.3_0.1/1, FrontObj_Line_0.8_0.8/1
  [K] -> Index Vector3/1
  Assignment1/1 -> obj_Front_sub_DPC/1
  Constant1/1 -> Assignment1/1
  [K] -> Assignment1/3
  [K] -> Index Vector2/1
  Assignment/1 -> obj_Rear_sub_DPC/1
  [K] -> Assignment/3
  Constant3/1 -> Assignment/1
  [K] -> Index Vector4/1
  For Iterator/1 -> [K], Index Vector/1
  obj_Rear_Vx/1 -> Index Vector/2
  Rearobj_Line_0.3_0.3/1 -> Mux/2  "Rearobj_Line_0.3"
  Index Vector/1 -> Rearobj_Line_0_0/1, Rearobj_Line_1_1/1, Rearobj_Line_0.8_0.8/1, Rearobj_Line_0.3_0.3/1
  Mux1/1 -> Data Type Conversion3/1
  FrontObj_Line_0.8_0.8/1 -> Mux1/2  "FrontObj_Line_0.8"
  obj_Front_sub_Dx/1 -> Index Vector2/2
  FrontObj_Line_1_1/1 -> Mux1/1  "FrontObj_Line_1"
  1-D Lookup Table1/1 -> Saturation1/1
  Rearobj_Line_1_1/1 -> Mux/4  "Rearobj_Line_1"
  FrontObj_Line_0_1/1 -> Mux1/4  "FrontObj_Line_0"
  1-D Lookup Table8/1 -> Saturation/1
  Mux/1 -> Data Type Conversion5/1
  obj_Rear_sub_Dx/1 -> Index Vector4/2
  Rearobj_Line_0_0/1 -> Mux/1  "Rearobj_Line_0"
  FrontObj_Line_0.3_0.1/1 -> Mux1/3  "FrontObj_Line_0.3"
  Rearobj_Line_0.8_0.8/1 -> Mux/3  "Rearobj_Line_0.8"
  Constant/1 -> FrontObj_Line_1_1/3
  Constant2/1 -> FrontObj_Line_1_1/2
  Constant4/1 -> FrontObj_Line_0.8_0.8/3
  Constant5/1 -> FrontObj_Line_0.8_0.8/2
  Constant6/1 -> FrontObj_Line_0.3_0.1/3
  Constant7/1 -> FrontObj_Line_0.3_0.1/2
  Constant8/1 -> FrontObj_Line_0_1/3
  Constant9/1 -> FrontObj_Line_0_1/2
  Constant11/1 -> Rearobj_Line_0_0/2
  Constant10/1 -> Rearobj_Line_0_0/3
  Constant13/1 -> Rearobj_Line_0.3_0.3/2
  Constant12/1 -> Rearobj_Line_0.3_0.3/3
  Constant14/1 -> Rearobj_Line_0.8_0.8/3
  Constant15/1 -> Rearobj_Line_0.8_0.8/2
  Constant17/1 -> Rearobj_Line_1_1/2
  Constant16/1 -> Rearobj_Line_1_1/3

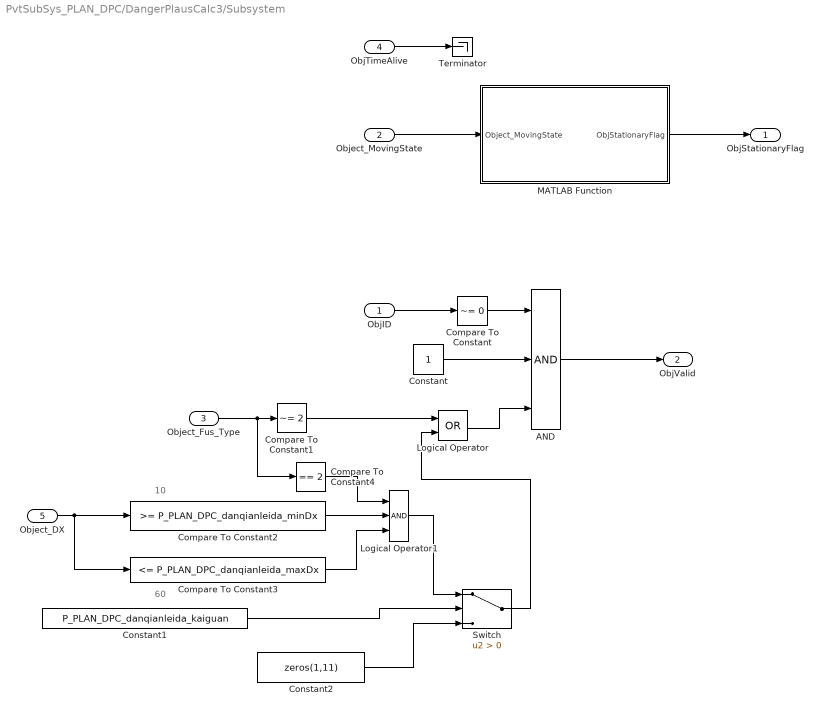
== system PvtSubSys_PLAN_DPC/DangerPlausCalc3/Subsystem ==
  note: 10
  note: 60
  ObjID : Inport
  Object_MovingState : Inport  Port=2
  Object_Fus_Type : Inport  Port=3
  ObjTimeAlive : Inport  Port=4
  Object_DX : Inport  Port=5
  AND : Logic  Inputs=3  AllPortsSameDT=off  OutDataTypeStr=boolean
  Compare To Constant : simulink/Logic and Bit Operations/Compare To Constant  relop=~=  const=0  OutDataTypeStr=boolean
  Compare To Constant1 : simulink/Logic and Bit Operations/Compare To Constant  relop=~=  const=2  OutDataTypeStr=boolean
  Compare To Constant2 : simulink/Logic and Bit Operations/Compare To Constant  relop=>=  const=P_PLAN_DPC_danqianleida_minDx  OutDataTypeStr=boolean
  Compare To Constant3 : simulink/Logic and Bit Operations/Compare To Constant  relop=<=  const=P_PLAN_DPC_danqianleida_maxDx  OutDataTypeStr=boolean
  Compare To Constant4 : simulink/Logic and Bit Operations/Compare To Constant  relop===  const=2  OutDataTypeStr=boolean
  Constant : Constant
  Constant1 : Constant  Value=P_PLAN_DPC_danqianleida_kaiguan
  Constant2 : Constant  Value=zeros(1,11)
  Logical Operator : Logic  Operator=OR  AllPortsSameDT=off  OutDataTypeStr=boolean
  Logical Operator1 : Logic  Inputs=3  AllPortsSameDT=off  OutDataTypeStr=boolean
  MATLAB Function : MATLAB Function  TreatAsAtomicUnit=on
  Switch : Switch  Criteria=u2 > Threshold
  Terminator : Terminator
  ObjStationaryFlag : Outport
  ObjValid : Outport  Port=2
  wires:
  Constant2/1 -> Switch/3
  Constant1/1 -> Switch/2
  Switch/1 -> Logical Operator/2
  Logical Operator1/1 -> Switch/1
  Logical Operator/1 -> AND/3
  Compare To Constant4/1 -> Logical Operator1/1
  Compare To Constant3/1 -> Logical Operator1/3
  Compare To Constant2/1 -> Logical Operator1/2
  Object_DX/1 -> Compare To Constant2/1, Compare To Constant3/1
  Compare To Constant1/1 -> Logical Operator/1
  AND/1 -> ObjValid/1
  Compare To Constant/1 -> AND/1
  Constant/1 -> AND/2
  ObjID/1 -> Compare To Constant/1
  Object_Fus_Type/1 -> Compare To Constant1/1, Compare To Constant4/1
  ObjTimeAlive/1 -> Terminator/1
  MATLAB Function/1(ObjStationaryFlag) -> ObjStationaryFlag/1
  Object_MovingState/1 -> MATLAB Function/1(Object_MovingState)

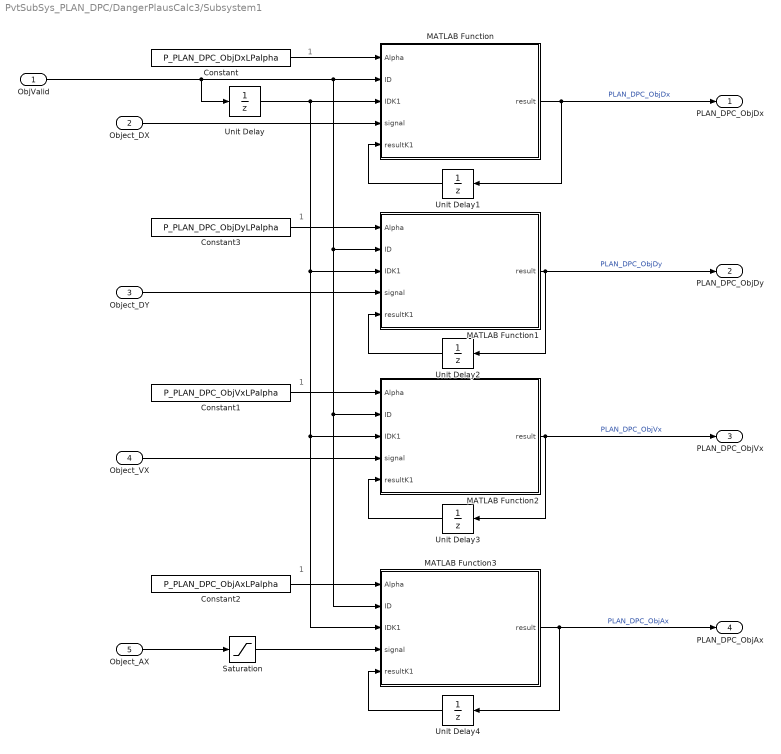
== system PvtSubSys_PLAN_DPC/DangerPlausCalc3/Subsystem1 ==
  note: 1
  note: 1
  note: 1
  note: 1
  ObjValid : Inport
  Object_DX : Inport  Port=2
  Object_DY : Inport  Port=3
  Object_VX : Inport  Port=4
  Object_AX : Inport  Port=5
  Constant : Constant  Value=P_PLAN_DPC_ObjDxLPalpha
  Constant1 : Constant  Value=P_PLAN_DPC_ObjVxLPalpha
  Constant2 : Constant  Value=P_PLAN_DPC_ObjAxLPalpha
  Constant3 : Constant  Value=P_PLAN_DPC_ObjDyLPalpha
  MATLAB Function : MATLAB Function  TreatAsAtomicUnit=on
  MATLAB Function1 : MATLAB Function  TreatAsAtomicUnit=on
  MATLAB Function2 : MATLAB Function  TreatAsAtomicUnit=on
  MATLAB Function3 : MATLAB Function  TreatAsAtomicUnit=on
  Saturation : Saturate  UpperLimit=4  LowerLimit=-4
  Unit Delay{,1..4} (5 alike) : UnitDelay  SampleTime=-1  HasFrameUpgradeWarning=on
  PLAN_DPC_ObjDx : Outport
  PLAN_DPC_ObjDy : Outport  Port=2
  PLAN_DPC_ObjVx : Outport  Port=3
  PLAN_DPC_ObjAx : Outport  Port=4
  wires:
  Saturation/1 -> MATLAB Function3/4(signal)
  Constant2/1 -> MATLAB Function3/1(Alpha)
  MATLAB Function3/1(result) -> Unit Delay4/1, PLAN_DPC_ObjAx/1  "PLAN_DPC_ObjAx"
  Object_AX/1 -> Saturation/1
  Unit Delay4/1 -> MATLAB Function3/5(resultK1)
  Constant1/1 -> MATLAB Function2/1(Alpha)
  Constant3/1 -> MATLAB Function1/1(Alpha)
  Constant/1 -> MATLAB Function/1(Alpha)
  Unit Delay3/1 -> MATLAB Function2/5(resultK1)
  MATLAB Function2/1(result) -> Unit Delay3/1, PLAN_DPC_ObjVx/1  "PLAN_DPC_ObjVx"
  MATLAB Function1/1(result) -> Unit Delay2/1, PLAN_DPC_ObjDy/1  "PLAN_DPC_ObjDy"
  Unit Delay2/1 -> MATLAB Function1/5(resultK1)
  ObjValid/1 -> MATLAB Function/2(ID), MATLAB Function1/2(ID), MATLAB Function3/2(ID), MATLAB Function2/2(ID), Unit Delay/1
  Object_DX/1 -> MATLAB Function/4(signal)
  Unit Delay/1 -> MATLAB Function/3(IDK1), MATLAB Function1/3(IDK1), MATLAB Function3/3(IDK1), MATLAB Function2/3(IDK1)
  Unit Delay1/1 -> MATLAB Function/5(resultK1)
  Object_DY/1 -> MATLAB Function1/4(signal)
  Object_VX/1 -> MATLAB Function2/4(signal)
  MATLAB Function/1(result) -> PLAN_DPC_ObjDx/1, Unit Delay1/1  "PLAN_DPC_ObjDx"
